simulink model "WorkingModel"  (R2023b)
settings: Solver=FixedStepDiscrete  StartTime=0.0  StopTime=param_sim_time  FixedStep=1/fs  MaxStep=1/fs  RelTol=1e-3
undefined symbols (not defined in the file): analyses, fdesignblkfcn, fs, gcbh, param_tot_samples
libraries: dspstat3 x13, SCGAnalysis_SignalGenerationLib x2
(part 9 of 20)

== system WorkingModel/SCG Analysis/Enabled SCG Analysis Subsystem/All Signals Signal Metric Characterization/SCG Systolic 3DMinS1p2pProjection Signal Metric Characterization/Average Cycle-to-cycle Morphological Variability Calculator ==
  note: This subsystem is only enabled when its signal metric flag is raised.
  in_r_pos : Inport
  in_scg_signal : Inport  Port=2
  Enable : EnablePort
  Average Cycle-to-cycle Morphological Variability Calculator : MATLAB Function  TreatAsAtomicUnit=on
  Constant : Constant  Value=fs
  out_morphological_variability : Outport
  wires:
  Constant/1 -> Average Cycle-to-cycle Morphological Variability Calculator/1(fs)
  Average Cycle-to-cycle Morphological Variability Calculator/1(variability) -> out_morphological_variability/1
  in_scg_signal/1 -> Average Cycle-to-cycle Morphological Variability Calculator/3(scg_signal)
  in_r_pos/1 -> Average Cycle-to-cycle Morphological Variability Calculator/2(r_pos)

== system WorkingModel/SCG Analysis/Enabled SCG Analysis Subsystem/All Signals Signal Metric Characterization/SCG Systolic 3DMinS1p2pProjection Signal Metric Characterization/Average S1 peak-to-peak Amplitude Calculator ==
  note: This subsystem is only enabled when its signal metric flag is raised.
  in_r_pos : Inport
  in_scg_sig : Inport  Port=2
  Enable : EnablePort
  Average S1p2p Amplitude Calculator : MATLAB Function  TreatAsAtomicUnit=on
  Constant : Constant  Value=fs
  out_average_s1p2pamp : Outport
  wires:
  Constant/1 -> Average S1p2p Amplitude Calculator/1(fs)
  in_r_pos/1 -> Average S1p2p Amplitude Calculator/2(r_pos)
  Average S1p2p Amplitude Calculator/1(average_s1p2pamp) -> out_average_s1p2pamp/1
  in_scg_sig/1 -> Average S1p2p Amplitude Calculator/3(scg_signal)

== system WorkingModel/SCG Analysis/Enabled SCG Analysis Subsystem/All Signals Signal Metric Characterization/SCG Systolic 3DMinS1p2pProjection Signal Metric Characterization/Average S2 peak-to-peak Amplitude Calculator ==
  note: This subsystem is only enabled when its signal metric flag is raised.
  in_r_pos : Inport
  in_scg_signal : Inport  Port=2
  Enable : EnablePort
  Average S2p2p Amplitude Calculator : MATLAB Function  TreatAsAtomicUnit=on
  Constant : Constant  Value=fs
  out_scg_signal_average_s2p2pamp : Outport
  wires:
  in_scg_signal/1 -> Average S2p2p Amplitude Calculator/3(scg_signal)
  Average S2p2p Amplitude Calculator/1(average_s2p2pamp) -> out_scg_signal_average_s2p2pamp/1
  in_r_pos/1 -> Average S2p2p Amplitude Calculator/2(r_pos)
  Constant/1 -> Average S2p2p Amplitude Calculator/1(fs)

== system WorkingModel/SCG Analysis/Enabled SCG Analysis Subsystem/All Signals Signal Metric Characterization/SCG Systolic 3DMinS1p2pProjection Signal Metric Characterization/Average Signal-to-Noise Ratio Calculator ==
  note: This subsystem is only enabled when its signal metric flag is raised.
  in_r_pos : Inport
  in_scg_signal : Inport  Port=2
  Enable : EnablePort  PropagateVarSize=During execution
  Average S1 Signal-to-Noise Ratio : Subsystem
  Average S1X Signal-to-Noise Ratio : Subsystem
  Average S2 Signal-to-Noise Ratio : Subsystem
  Average S2X Signal-to-Noise Ratio : Subsystem
  out_scg_signal_average_s1snr : Outport
  out_scg_signal_average_s1Xsnr : Outport  Port=2
  out_scg_signal_average_s2snr : Outport  Port=3
  out_scg_signal_average_s2Xsnr : Outport  Port=4
  wires:
  Average S2X Signal-to-Noise Ratio/1(average_s2Xsnr) -> out_scg_signal_average_s2Xsnr/1
  in_r_pos/1 -> Average S1 Signal-to-Noise Ratio/1(r_pos), Average S2X Signal-to-Noise Ratio/1(r_pos), Average S2 Signal-to-Noise Ratio/1(r_pos), Average S1X Signal-to-Noise Ratio/1(r_pos)
  Average S2 Signal-to-Noise Ratio/1(average_s2snr) -> out_scg_signal_average_s2snr/1
  Average S1X Signal-to-Noise Ratio/1(average_s1Xsnr) -> out_scg_signal_average_s1Xsnr/1
  in_scg_signal/1 -> Average S2X Signal-to-Noise Ratio/2(scg_signal), Average S2 Signal-to-Noise Ratio/2(scg_signal), Average S1X Signal-to-Noise Ratio/2(scg_signal), Average S1 Signal-to-Noise Ratio/2(scg_signal)
  Average S1 Signal-to-Noise Ratio/1(average_s1snr) -> out_scg_signal_average_s1snr/1

== system WorkingModel/SCG Analysis/Enabled SCG Analysis Subsystem/All Signals Signal Metric Characterization/SCG Systolic 3DMinS1p2pProjection Signal Metric Characterization/Spectral Distribution Calculator ==
  note: This subsystem is only enabled when its signal metric flag is raised.
  in_r_pos : Inport
  in_scg_signal : Inport  Port=2
  Enable : EnablePort
  Constant : Constant  Value=fs
  Constant1 : Constant  Value=entire_cycle
  Constant2 : Constant  Value=s1
  Constant3 : Constant  Value=s2
  Constant4 : Constant  Value=f_band_lo
  Constant5 : Constant  Value=f_band_mid
  Constant6 : Constant  Value=f_band_hi
  Spectral Distribution Calculator : MATLAB Function  TreatAsAtomicUnit=on
  out_entire_cycle_spectral_distribution : Outport
  out_s1_spectral_distribution : Outport  Port=2
  out_s2_spectral_distribution : Outport  Port=3
  wires:
  in_r_pos/1 -> Spectral Distribution Calculator/2(r_pos)
  in_scg_signal/1 -> Spectral Distribution Calculator/3(scg_signal)
  Spectral Distribution Calculator/1(entire_cycle_nsd) -> out_entire_cycle_spectral_distribution/1
  Constant/1 -> Spectral Distribution Calculator/1(fs)
  Constant1/1 -> Spectral Distribution Calculator/4(entire_cycle_flag)
  Constant4/1 -> Spectral Distribution Calculator/7(f_band_lo)
  Constant6/1 -> Spectral Distribution Calculator/9(f_band_hi)
  Constant5/1 -> Spectral Distribution Calculator/8(f_band_mid)
  Constant3/1 -> Spectral Distribution Calculator/6(s2_flag)
  Constant2/1 -> Spectral Distribution Calculator/5(s1_flag)
  Spectral Distribution Calculator/3(s2_nsd) -> out_s2_spectral_distribution/1
  Spectral Distribution Calculator/2(s1_nsd) -> out_s1_spectral_distribution/1

== system WorkingModel/SCG Analysis/Enabled SCG Analysis Subsystem/All Signals Signal Metric Characterization/SCG Systolic 3DMinS1p2pProjection Signal Metric Characterization/Variance ==
  note: This subsystem is only enabled when its signal metric flag is raised.
  in_scg_signal : Inport
  Enable : EnablePort
  Variance : dspstat3/Variance  run=off  InputProcessing=Columns as channels (frame based)  reset_popup=None  directionMode=Each column  dimension=1  roiEnable=off  roiType=Rectangles  roiPortion=Entire ROI  roiOutput=Individual statistics for each ROI  roiFlag=off  roundingMode=Floor  overflowMode=off
  out_scg_signal_var : Outport
  wires:
  Variance/1 -> out_scg_signal_var/1
  in_scg_signal/1 -> Variance/1

== system WorkingModel/SCG Analysis/Enabled SCG Analysis Subsystem/All Signals Signal Metric Characterization/SCG X Signal Metric Characterization/Average Cycle-to-cycle Morphological Variability Calculator ==
  note: This subsystem is only enabled when its signal metric flag is raised.
  in_r_pos : Inport
  in_scg_signal : Inport  Port=2
  Enable : EnablePort
  Average Cycle-to-cycle Morphological Variability Calculator : MATLAB Function  TreatAsAtomicUnit=on
  Constant : Constant  Value=fs
  out_morphological_variability : Outport
  wires:
  Constant/1 -> Average Cycle-to-cycle Morphological Variability Calculator/1(fs)
  Average Cycle-to-cycle Morphological Variability Calculator/1(variability) -> out_morphological_variability/1
  in_scg_signal/1 -> Average Cycle-to-cycle Morphological Variability Calculator/3(scg_signal)
  in_r_pos/1 -> Average Cycle-to-cycle Morphological Variability Calculator/2(r_pos)

== system WorkingModel/SCG Analysis/Enabled SCG Analysis Subsystem/All Signals Signal Metric Characterization/SCG X Signal Metric Characterization/Average S1 peak-to-peak Amplitude Calculator ==
  note: This subsystem is only enabled when its signal metric flag is raised.
  in_r_pos : Inport
  in_scg_sig : Inport  Port=2
  Enable : EnablePort
  Average S1p2p Amplitude Calculator : MATLAB Function  TreatAsAtomicUnit=on
  Constant : Constant  Value=fs
  out_average_s1p2pamp : Outport
  wires:
  Constant/1 -> Average S1p2p Amplitude Calculator/1(fs)
  in_r_pos/1 -> Average S1p2p Amplitude Calculator/2(r_pos)
  Average S1p2p Amplitude Calculator/1(average_s1p2pamp) -> out_average_s1p2pamp/1
  in_scg_sig/1 -> Average S1p2p Amplitude Calculator/3(scg_signal)

== system WorkingModel/SCG Analysis/Enabled SCG Analysis Subsystem/All Signals Signal Metric Characterization/SCG X Signal Metric Characterization/Average S2 peak-to-peak Amplitude Calculator ==
  note: This subsystem is only enabled when its signal metric flag is raised.
  in_r_pos : Inport
  in_scg_signal : Inport  Port=2
  Enable : EnablePort
  Average S2p2p Amplitude Calculator : MATLAB Function  TreatAsAtomicUnit=on
  Constant : Constant  Value=fs
  out_scg_signal_average_s2p2pamp : Outport
  wires:
  in_scg_signal/1 -> Average S2p2p Amplitude Calculator/3(scg_signal)
  Average S2p2p Amplitude Calculator/1(average_s2p2pamp) -> out_scg_signal_average_s2p2pamp/1
  in_r_pos/1 -> Average S2p2p Amplitude Calculator/2(r_pos)
  Constant/1 -> Average S2p2p Amplitude Calculator/1(fs)

== system WorkingModel/SCG Analysis/Enabled SCG Analysis Subsystem/All Signals Signal Metric Characterization/SCG X Signal Metric Characterization/Average Signal-to-Noise Ratio Calculator ==
  note: This subsystem is only enabled when its signal metric flag is raised.
  in_r_pos : Inport
  in_scg_signal : Inport  Port=2
  Enable : EnablePort  PropagateVarSize=During execution
  Average S1 Signal-to-Noise Ratio : Subsystem
  Average S1X Signal-to-Noise Ratio : Subsystem
  Average S2 Signal-to-Noise Ratio : Subsystem
  Average S2X Signal-to-Noise Ratio : Subsystem
  out_scg_signal_average_s1snr : Outport
  out_scg_signal_average_s1Xsnr : Outport  Port=2
  out_scg_signal_average_s2snr : Outport  Port=3
  out_scg_signal_average_s2Xsnr : Outport  Port=4
  wires:
  Average S2X Signal-to-Noise Ratio/1(average_s2Xsnr) -> out_scg_signal_average_s2Xsnr/1
  in_r_pos/1 -> Average S1 Signal-to-Noise Ratio/1(r_pos), Average S2X Signal-to-Noise Ratio/1(r_pos), Average S2 Signal-to-Noise Ratio/1(r_pos), Average S1X Signal-to-Noise Ratio/1(r_pos)
  Average S2 Signal-to-Noise Ratio/1(average_s2snr) -> out_scg_signal_average_s2snr/1
  Average S1X Signal-to-Noise Ratio/1(average_s1Xsnr) -> out_scg_signal_average_s1Xsnr/1
  in_scg_signal/1 -> Average S2X Signal-to-Noise Ratio/2(scg_signal), Average S2 Signal-to-Noise Ratio/2(scg_signal), Average S1X Signal-to-Noise Ratio/2(scg_signal), Average S1 Signal-to-Noise Ratio/2(scg_signal)
  Average S1 Signal-to-Noise Ratio/1(average_s1snr) -> out_scg_signal_average_s1snr/1

== system WorkingModel/SCG Analysis/Enabled SCG Analysis Subsystem/All Signals Signal Metric Characterization/SCG X Signal Metric Characterization/Spectral Distribution Calculator ==
  note: This subsystem is only enabled when its signal metric flag is raised.
  in_r_pos : Inport
  in_scg_signal : Inport  Port=2
  Enable : EnablePort
  Constant : Constant  Value=fs
  Constant1 : Constant  Value=entire_cycle
  Constant2 : Constant  Value=s1
  Constant3 : Constant  Value=s2
  Constant4 : Constant  Value=f_band_lo
  Constant5 : Constant  Value=f_band_mid
  Constant6 : Constant  Value=f_band_hi
  Spectral Distribution Calculator : MATLAB Function  TreatAsAtomicUnit=on
  out_entire_cycle_spectral_distribution : Outport
  out_s1_spectral_distribution : Outport  Port=2
  out_s2_spectral_distribution : Outport  Port=3
  wires:
  in_r_pos/1 -> Spectral Distribution Calculator/2(r_pos)
  in_scg_signal/1 -> Spectral Distribution Calculator/3(scg_signal)
  Spectral Distribution Calculator/1(entire_cycle_nsd) -> out_entire_cycle_spectral_distribution/1
  Constant/1 -> Spectral Distribution Calculator/1(fs)
  Constant1/1 -> Spectral Distribution Calculator/4(entire_cycle_flag)
  Constant4/1 -> Spectral Distribution Calculator/7(f_band_lo)
  Constant6/1 -> Spectral Distribution Calculator/9(f_band_hi)
  Constant5/1 -> Spectral Distribution Calculator/8(f_band_mid)
  Constant3/1 -> Spectral Distribution Calculator/6(s2_flag)
  Constant2/1 -> Spectral Distribution Calculator/5(s1_flag)
  Spectral Distribution Calculator/3(s2_nsd) -> out_s2_spectral_distribution/1
  Spectral Distribution Calculator/2(s1_nsd) -> out_s1_spectral_distribution/1

== system WorkingModel/SCG Analysis/Enabled SCG Analysis Subsystem/All Signals Signal Metric Characterization/SCG X Signal Metric Characterization/Variance ==
  note: This subsystem is only enabled when its signal metric flag is raised.
  in_scg_signal : Inport
  Enable : EnablePort
  Variance : dspstat3/Variance  run=off  InputProcessing=Columns as channels (frame based)  reset_popup=None  directionMode=Each column  dimension=1  roiEnable=off  roiType=Rectangles  roiPortion=Entire ROI  roiOutput=Individual statistics for each ROI  roiFlag=off  roundingMode=Floor  overflowMode=off
  out_scg_signal_var : Outport
  wires:
  Variance/1 -> out_scg_signal_var/1
  in_scg_signal/1 -> Variance/1

== system WorkingModel/SCG Analysis/Enabled SCG Analysis Subsystem/All Signals Signal Metric Characterization/SCG Y Signal Metric Characterization/Average Cycle-to-cycle Morphological Variability Calculator ==
  note: This subsystem is only enabled when its signal metric flag is raised.
  in_r_pos : Inport
  in_scg_signal : Inport  Port=2
  Enable : EnablePort
  Average Cycle-to-cycle Morphological Variability Calculator : MATLAB Function  TreatAsAtomicUnit=on
  Constant : Constant  Value=fs
  out_morphological_variability : Outport
  wires:
  in_r_pos/1 -> Average Cycle-to-cycle Morphological Variability Calculator/2(r_pos)
  in_scg_signal/1 -> Average Cycle-to-cycle Morphological Variability Calculator/3(scg_signal)
  Average Cycle-to-cycle Morphological Variability Calculator/1(variability) -> out_morphological_variability/1
  Constant/1 -> Average Cycle-to-cycle Morphological Variability Calculator/1(fs)

== system WorkingModel/SCG Analysis/Enabled SCG Analysis Subsystem/All Signals Signal Metric Characterization/SCG Y Signal Metric Characterization/Average S1 peak-to-peak Amplitude Calculator ==
  note: This subsystem is only enabled when its signal metric flag is raised.
  in_r_pos : Inport
  in_scg_sig : Inport  Port=2
  Enable : EnablePort
  Average S1p2p Amplitude Calculator : MATLAB Function  TreatAsAtomicUnit=on
  Constant : Constant  Value=fs
  out_average_s1p2pamp : Outport
  wires:
  in_scg_sig/1 -> Average S1p2p Amplitude Calculator/3(scg_signal)
  Average S1p2p Amplitude Calculator/1(average_s1p2pamp) -> out_average_s1p2pamp/1
  in_r_pos/1 -> Average S1p2p Amplitude Calculator/2(r_pos)
  Constant/1 -> Average S1p2p Amplitude Calculator/1(fs)

== system WorkingModel/SCG Analysis/Enabled SCG Analysis Subsystem/All Signals Signal Metric Characterization/SCG Y Signal Metric Characterization/Average S2 peak-to-peak Amplitude Calculator ==
  note: This subsystem is only enabled when its signal metric flag is raised.
  in_r_pos : Inport
  in_scg_signal : Inport  Port=2
  Enable : EnablePort
  Average S2p2p Amplitude Calculator : MATLAB Function  TreatAsAtomicUnit=on
  Constant : Constant  Value=fs
  out_scg_signal_average_s2p2pamp : Outport
  wires:
  Constant/1 -> Average S2p2p Amplitude Calculator/1(fs)
  in_r_pos/1 -> Average S2p2p Amplitude Calculator/2(r_pos)
  Average S2p2p Amplitude Calculator/1(average_s2p2pamp) -> out_scg_signal_average_s2p2pamp/1
  in_scg_signal/1 -> Average S2p2p Amplitude Calculator/3(scg_signal)

== system WorkingModel/SCG Analysis/Enabled SCG Analysis Subsystem/All Signals Signal Metric Characterization/SCG Y Signal Metric Characterization/Average Signal-to-Noise Ratio Calculator ==
  note: This subsystem is only enabled when its signal metric flag is raised.
  in_r_pos : Inport
  in_scg_signal : Inport  Port=2
  Enable : EnablePort  PropagateVarSize=During execution
  Average S1 Signal-to-Noise Ratio : Subsystem
  Average S1X Signal-to-Noise Ratio : Subsystem
  Average S2 Signal-to-Noise Ratio : Subsystem
  Average S2X Signal-to-Noise Ratio : Subsystem
  out_scg_signal_average_s1snr : Outport
  out_scg_signal_average_s1Xsnr : Outport  Port=2
  out_scg_signal_average_s2snr : Outport  Port=3
  out_scg_signal_average_s2Xsnr : Outport  Port=4
  wires:
  Average S1 Signal-to-Noise Ratio/1(average_s1snr) -> out_scg_signal_average_s1snr/1
  in_scg_signal/1 -> Average S1 Signal-to-Noise Ratio/2(scg_signal), Average S1X Signal-to-Noise Ratio/2(scg_signal), Average S2 Signal-to-Noise Ratio/2(scg_signal), Average S2X Signal-to-Noise Ratio/2(scg_signal)
  Average S1X Signal-to-Noise Ratio/1(average_s1Xsnr) -> out_scg_signal_average_s1Xsnr/1
  Average S2 Signal-to-Noise Ratio/1(average_s2snr) -> out_scg_signal_average_s2snr/1
  in_r_pos/1 -> Average S1X Signal-to-Noise Ratio/1(r_pos), Average S2 Signal-to-Noise Ratio/1(r_pos), Average S2X Signal-to-Noise Ratio/1(r_pos), Average S1 Signal-to-Noise Ratio/1(r_pos)
  Average S2X Signal-to-Noise Ratio/1(average_s2Xsnr) -> out_scg_signal_average_s2Xsnr/1

== system WorkingModel/SCG Analysis/Enabled SCG Analysis Subsystem/All Signals Signal Metric Characterization/SCG Y Signal Metric Characterization/Spectral Distribution Calculator ==
  note: This subsystem is only enabled when its signal metric flag is raised.
  in_r_pos : Inport
  in_scg_signal : Inport  Port=2
  Enable : EnablePort
  Constant : Constant  Value=fs
  Constant1 : Constant  Value=entire_cycle
  Constant2 : Constant  Value=s1
  Constant3 : Constant  Value=s2
  Constant4 : Constant  Value=f_band_lo
  Constant5 : Constant  Value=f_band_mid
  Constant6 : Constant  Value=f_band_hi
  Spectral Distribution Calculator : MATLAB Function  TreatAsAtomicUnit=on
  out_entire_cycle_spectral_distribution : Outport
  out_s1_spectral_distribution : Outport  Port=2
  out_s2_spectral_distribution : Outport  Port=3
  wires:
  Spectral Distribution Calculator/2(s1_nsd) -> out_s1_spectral_distribution/1
  Spectral Distribution Calculator/3(s2_nsd) -> out_s2_spectral_distribution/1
  Constant2/1 -> Spectral Distribution Calculator/5(s1_flag)
  Constant3/1 -> Spectral Distribution Calculator/6(s2_flag)
  Constant5/1 -> Spectral Distribution Calculator/8(f_band_mid)
  Constant6/1 -> Spectral Distribution Calculator/9(f_band_hi)
  Constant4/1 -> Spectral Distribution Calculator/7(f_band_lo)
  Constant1/1 -> Spectral Distribution Calculator/4(entire_cycle_flag)
  Constant/1 -> Spectral Distribution Calculator/1(fs)
  Spectral Distribution Calculator/1(entire_cycle_nsd) -> out_entire_cycle_spectral_distribution/1
  in_scg_signal/1 -> Spectral Distribution Calculator/3(scg_signal)
  in_r_pos/1 -> Spectral Distribution Calculator/2(r_pos)

== system WorkingModel/SCG Analysis/Enabled SCG Analysis Subsystem/All Signals Signal Metric Characterization/SCG Y Signal Metric Characterization/Variance ==
  note: This subsystem is only enabled when its signal metric flag is raised.
  in_scg_signal : Inport
  Enable : EnablePort
  Variance : dspstat3/Variance  run=off  InputProcessing=Columns as channels (frame based)  reset_popup=None  directionMode=Each column  dimension=1  roiEnable=off  roiType=Rectangles  roiPortion=Entire ROI  roiOutput=Individual statistics for each ROI  roiFlag=off  roundingMode=Floor  overflowMode=off
  out_scg_signal_var : Outport
  wires:
  in_scg_signal/1 -> Variance/1
  Variance/1 -> out_scg_signal_var/1

== system WorkingModel/SCG Analysis/Enabled SCG Analysis Subsystem/All Signals Signal Metric Characterization/SCG Z Signal Metric Characterization/Average Cycle-to-cycle Morphological Variability Calculator ==
  note: This subsystem is only enabled when its signal metric flag is raised.
  in_r_pos : Inport
  in_scg_signal : Inport  Port=2
  Enable : EnablePort
  Average Cycle-to-cycle Morphological Variability Calculator : MATLAB Function  TreatAsAtomicUnit=on
  Constant : Constant  Value=fs
  out_morphological_variability : Outport
  wires:
  Constant/1 -> Average Cycle-to-cycle Morphological Variability Calculator/1(fs)
  Average Cycle-to-cycle Morphological Variability Calculator/1(variability) -> out_morphological_variability/1
  in_scg_signal/1 -> Average Cycle-to-cycle Morphological Variability Calculator/3(scg_signal)
  in_r_pos/1 -> Average Cycle-to-cycle Morphological Variability Calculator/2(r_pos)

== system WorkingModel/SCG Analysis/Enabled SCG Analysis Subsystem/All Signals Signal Metric Characterization/SCG Z Signal Metric Characterization/Average S1 peak-to-peak Amplitude Calculator ==
  note: This subsystem is only enabled when its signal metric flag is raised.
  in_r_pos : Inport
  in_scg_sig : Inport  Port=2
  Enable : EnablePort
  Average S1p2p Amplitude Calculator : MATLAB Function  TreatAsAtomicUnit=on
  Constant : Constant  Value=fs
  out_average_s1p2pamp : Outport
  wires:
  Constant/1 -> Average S1p2p Amplitude Calculator/1(fs)
  in_r_pos/1 -> Average S1p2p Amplitude Calculator/2(r_pos)
  Average S1p2p Amplitude Calculator/1(average_s1p2pamp) -> out_average_s1p2pamp/1
  in_scg_sig/1 -> Average S1p2p Amplitude Calculator/3(scg_signal)

== system WorkingModel/SCG Analysis/Enabled SCG Analysis Subsystem/All Signals Signal Metric Characterization/SCG Z Signal Metric Characterization/Average S2 peak-to-peak Amplitude Calculator ==
  note: This subsystem is only enabled when its signal metric flag is raised.
  in_r_pos : Inport
  in_scg_signal : Inport  Port=2
  Enable : EnablePort
  Average S2p2p Amplitude Calculator : MATLAB Function  TreatAsAtomicUnit=on
  Constant : Constant  Value=fs
  out_scg_signal_average_s2p2pamp : Outport
  wires:
  in_scg_signal/1 -> Average S2p2p Amplitude Calculator/3(scg_signal)
  Average S2p2p Amplitude Calculator/1(average_s2p2pamp) -> out_scg_signal_average_s2p2pamp/1
  in_r_pos/1 -> Average S2p2p Amplitude Calculator/2(r_pos)
  Constant/1 -> Average S2p2p Amplitude Calculator/1(fs)

== system WorkingModel/SCG Analysis/Enabled SCG Analysis Subsystem/All Signals Signal Metric Characterization/SCG Z Signal Metric Characterization/Average Signal-to-Noise Ratio Calculator ==
  note: This subsystem is only enabled when its signal metric flag is raised.
  in_r_pos : Inport
  in_scg_signal : Inport  Port=2
  Enable : EnablePort  PropagateVarSize=During execution
  Average S1 Signal-to-Noise Ratio : Subsystem
  Average S1X Signal-to-Noise Ratio : Subsystem
  Average S2 Signal-to-Noise Ratio : Subsystem
  Average S2X Signal-to-Noise Ratio : Subsystem
  out_scg_signal_average_s1snr : Outport
  out_scg_signal_average_s1Xsnr : Outport  Port=2
  out_scg_signal_average_s2snr : Outport  Port=3
  out_scg_signal_average_s2Xsnr : Outport  Port=4
  wires:
  Average S2X Signal-to-Noise Ratio/1(average_s2Xsnr) -> out_scg_signal_average_s2Xsnr/1
  in_r_pos/1 -> Average S1 Signal-to-Noise Ratio/1(r_pos), Average S2X Signal-to-Noise Ratio/1(r_pos), Average S2 Signal-to-Noise Ratio/1(r_pos), Average S1X Signal-to-Noise Ratio/1(r_pos)
  Average S2 Signal-to-Noise Ratio/1(average_s2snr) -> out_scg_signal_average_s2snr/1
  Average S1X Signal-to-Noise Ratio/1(average_s1Xsnr) -> out_scg_signal_average_s1Xsnr/1
  in_scg_signal/1 -> Average S2X Signal-to-Noise Ratio/2(scg_signal), Average S2 Signal-to-Noise Ratio/2(scg_signal), Average S1X Signal-to-Noise Ratio/2(scg_signal), Average S1 Signal-to-Noise Ratio/2(scg_signal)
  Average S1 Signal-to-Noise Ratio/1(average_s1snr) -> out_scg_signal_average_s1snr/1

== system WorkingModel/SCG Analysis/Enabled SCG Analysis Subsystem/All Signals Signal Metric Characterization/SCG Z Signal Metric Characterization/Spectral Distribution Calculator ==
  note: This subsystem is only enabled when its signal metric flag is raised.
  in_r_pos : Inport
  in_scg_signal : Inport  Port=2
  Enable : EnablePort
  Constant : Constant  Value=fs
  Constant1 : Constant  Value=entire_cycle
  Constant2 : Constant  Value=s1
  Constant3 : Constant  Value=s2
  Constant4 : Constant  Value=f_band_lo
  Constant5 : Constant  Value=f_band_mid
  Constant6 : Constant  Value=f_band_hi
  Spectral Distribution Calculator : MATLAB Function  TreatAsAtomicUnit=on
  out_entire_cycle_spectral_distribution : Outport
  out_s1_spectral_distribution : Outport  Port=2
  out_s2_spectral_distribution : Outport  Port=3
  wires:
  in_r_pos/1 -> Spectral Distribution Calculator/2(r_pos)
  in_scg_signal/1 -> Spectral Distribution Calculator/3(scg_signal)
  Spectral Distribution Calculator/1(entire_cycle_nsd) -> out_entire_cycle_spectral_distribution/1
  Constant/1 -> Spectral Distribution Calculator/1(fs)
  Constant1/1 -> Spectral Distribution Calculator/4(entire_cycle_flag)
  Constant4/1 -> Spectral Distribution Calculator/7(f_band_lo)
  Constant6/1 -> Spectral Distribution Calculator/9(f_band_hi)
  Constant5/1 -> Spectral Distribution Calculator/8(f_band_mid)
  Constant3/1 -> Spectral Distribution Calculator/6(s2_flag)
  Constant2/1 -> Spectral Distribution Calculator/5(s1_flag)
  Spectral Distribution Calculator/3(s2_nsd) -> out_s2_spectral_distribution/1
  Spectral Distribution Calculator/2(s1_nsd) -> out_s1_spectral_distribution/1

== system WorkingModel/SCG Analysis/Enabled SCG Analysis Subsystem/All Signals Signal Metric Characterization/SCG Z Signal Metric Characterization/Variance ==
  note: This subsystem is only enabled when its signal metric flag is raised.
  in_scg_signal : Inport
  Enable : EnablePort
  Variance : dspstat3/Variance  run=off  InputProcessing=Columns as channels (frame based)  reset_popup=None  directionMode=Each column  dimension=1  roiEnable=off  roiType=Rectangles  roiPortion=Entire ROI  roiOutput=Individual statistics for each ROI  roiFlag=off  roundingMode=Floor  overflowMode=off
  out_scg_signal_var : Outport
  wires:
  Variance/1 -> out_scg_signal_var/1
  in_scg_signal/1 -> Variance/1

== system WorkingModel/SCG Analysis/Enabled SCG Analysis Subsystem/Signal Generation/2DMod Calculator/2DMod Calculator ==
  2D Components : Inport
  Square Root1 : Sqrt
  Square1 : Math  Operator=square  SignedPower=on
  Sum1 : Sum  Inputs=+  CollapseMode=Specified dimension  CollapseDim=2
  2D Modulus : Outport  VectorParamsAs1DForOutWhenUnconnected=off
  wires:
  Square1/1 -> Sum1/1
  Sum1/1 -> Square Root1/1
  2D Components/1 -> Square1/1
  Square Root1/1 -> 2D Modulus/1

== system WorkingModel/SCG Analysis/Enabled SCG Analysis Subsystem/Signal Generation/3D Projections/3D Max S2 p2p Axis Calculator ==
  avg_scg_xyz_s2 : Inport
  Max S2 P2P  Axis Finder 3D : MATLABFcn  MATLABFcn=cardiac_max_s2p2p_axis_finder_3D  OutputDimensions=4  Output1D=off
  Selector2 : Selector  InputPortWidth=4  IndexOptions=Index vector (dialog)  Indices=[1]  OutputSizes=1
  Selector3 : Selector  InputPortWidth=4  IndexOptions=Index vector (dialog)  Indices=[2]  OutputSizes=1
  Selector6 : Selector  InputPortWidth=4  IndexOptions=Index vector (dialog)  Indices=[3]  OutputSizes=1
  Selector7 : Selector  InputPortWidth=4  IndexOptions=Index vector (dialog)  Indices=[4]  OutputSizes=1
  out_max_s2_axis_elevation : Outport
  out_max_s2_axis_azimuth : Outport  Port=2
  out_min_s2_axis_elevation : Outport  Port=3
  out_min_s2_axis_azimuth : Outport  Port=4
  wires:
  avg_scg_xyz_s2/1 -> Max S2 P2P  Axis Finder 3D/1
  Max S2 P2P  Axis Finder 3D/1 -> Selector7/1, Selector6/1, Selector2/1, Selector3/1
  Selector2/1 -> out_max_s2_axis_elevation/1
  Selector3/1 -> out_max_s2_axis_azimuth/1
  Selector7/1 -> out_min_s2_axis_azimuth/1
  Selector6/1 -> out_min_s2_axis_elevation/1

== system WorkingModel/SCG Analysis/Enabled SCG Analysis Subsystem/Signal Generation/3D Projections/3D S2 Mechanical Axis Calculator ==
  in_avg_scg_xyz_s2 : Inport
  Cardiac Mechanical Diastolic Axis Finder 3D : MATLABFcn  MATLABFcn=cardiac_mech_diastolic_axis_finder_3D  OutputDimensions=4  Output1D=off
  Selector : Selector  InputPortWidth=4  IndexOptions=Index vector (dialog)  Indices=[1]  OutputSizes=1
  Selector1 : Selector  InputPortWidth=4  IndexOptions=Index vector (dialog)  Indices=[2]  OutputSizes=1
  Selector4 : Selector  InputPortWidth=4  IndexOptions=Index vector (dialog)  Indices=[3]  OutputSizes=1
  Selector5 : Selector  InputPortWidth=4  IndexOptions=Index vector (dialog)  Indices=[4]  OutputSizes=1
  out_s2_mech_axis_elevation : Outport
  out_s2_mech_axis_azimuth : Outport  Port=2
  out_s2_antimech_axis_elevation : Outport  Port=3
  out_s2_antimech_axis_azimuth : Outport  Port=4
  wires:
  in_avg_scg_xyz_s2/1 -> Cardiac Mechanical Diastolic Axis Finder 3D/1
  Selector1/1 -> out_s2_mech_axis_azimuth/1
  Selector4/1 -> out_s2_antimech_axis_elevation/1
  Selector/1 -> out_s2_mech_axis_elevation/1
  Selector5/1 -> out_s2_antimech_axis_azimuth/1
  Cardiac Mechanical Diastolic Axis Finder 3D/1 -> Selector1/1, Selector/1, Selector4/1, Selector5/1

== system WorkingModel/SCG Analysis/Enabled SCG Analysis Subsystem/Signal Generation/3D Projections/SCG xyz Average Cycle ==
  in_ecg_r : Inport
  in_scg_xyz : Inport  Port=2
  Average SCGxyz Cycle Calculator : MATLAB Function  TreatAsAtomicUnit=on
  Constant : Constant
  Fixed-Size Converter 2 : Selector  NumberOfDimensions=2  IndexOptions=Starting and ending indices (port),Index vector (dialog)  Indices=[1:min(analyses.ecg.RR)],[1 2 3]  OutputSizes=1,1
  Min RR Calculator : MATLAB Function  TreatAsAtomicUnit=on
  Mux : Mux  Inputs=2
  out_scg_xyz_avgcycle : Outport  VectorParamsAs1DForOutWhenUnconnected=off
  wires:
  in_scg_xyz/1 -> Average SCGxyz Cycle Calculator/2(scgxyz)
  in_ecg_r/1 -> Min RR Calculator/1(r_pos), Average SCGxyz Cycle Calculator/1(r_pos)
  Average SCGxyz Cycle Calculator/1(scgxyz_avgcycle) -> Fixed-Size Converter 2/1
  Fixed-Size Converter 2/1 -> out_scg_xyz_avgcycle/1
  Constant/1 -> Mux/1
  Min RR Calculator/1(min_rr) -> Mux/2
  Mux/1 -> Fixed-Size Converter 2/2

== system WorkingModel/SCG Analysis/Enabled SCG Analysis Subsystem/All Signals Signal Metric Characterization/SCG 2D Mod Signal Metric Characterization/Average Signal-to-Noise Ratio Calculator/Average S1 Signal-to-Noise Ratio ==
  r_pos : Inport
  scg_signal : Inport  Port=2
  " " : Constant  Value=s1snr_flag
  Average S1 SNR Calculator : MATLAB Function  TreatAsAtomicUnit=on
  Constant : Constant  Value=fs
  Constant1 : Constant  Value=0
  Switch : Switch  Criteria=u2 > Threshold  AllowDiffInputSizes=on  SaturateOnIntegerOverflow=off  InputSameDT=off
  average_s1snr : Outport
  wires:
  scg_signal/1 -> Average S1 SNR Calculator/3(scg_signal)
  Average S1 SNR Calculator/1(average_s1_snr) -> average_s1snr/1
  Constant/1 -> Average S1 SNR Calculator/1(fs)
  " "/1 -> Switch/2
  Switch/1 -> Average S1 SNR Calculator/2(r_pos)
  r_pos/1 -> Switch/1
  Constant1/1 -> Switch/3

== system WorkingModel/SCG Analysis/Enabled SCG Analysis Subsystem/All Signals Signal Metric Characterization/SCG 2D Mod Signal Metric Characterization/Average Signal-to-Noise Ratio Calculator/Average S1X Signal-to-Noise Ratio ==
  r_pos : Inport
  scg_signal : Inport  Port=2
  " " : Constant  Value=s1xsnr_flag
  Average S1 SNR Amplitude Calculator : MATLAB Function  TreatAsAtomicUnit=on
  Constant : Constant  Value=fs
  Constant1 : Constant  Value=0
  Switch : Switch  Criteria=u2 > Threshold  AllowDiffInputSizes=on  SaturateOnIntegerOverflow=off  InputSameDT=off
  average_s1Xsnr : Outport
  wires:
  Average S1 SNR Amplitude Calculator/1(average_s1x_snr) -> average_s1Xsnr/1
  Switch/1 -> Average S1 SNR Amplitude Calculator/2(r_pos)
  scg_signal/1 -> Average S1 SNR Amplitude Calculator/3(scg_signal)
  Constant/1 -> Average S1 SNR Amplitude Calculator/1(fs)
  " "/1 -> Switch/2
  Constant1/1 -> Switch/3
  r_pos/1 -> Switch/1

== system WorkingModel/SCG Analysis/Enabled SCG Analysis Subsystem/All Signals Signal Metric Characterization/SCG 2D Mod Signal Metric Characterization/Average Signal-to-Noise Ratio Calculator/Average S2 Signal-to-Noise Ratio ==
  r_pos : Inport
  scg_signal : Inport  Port=2
  " " : Constant  Value=s2snr_flag
  Average S2 SNR Calculator : MATLAB Function  TreatAsAtomicUnit=on
  Constant : Constant  Value=fs
  Constant1 : Constant  Value=0
  Switch : Switch  Criteria=u2 > Threshold  AllowDiffInputSizes=on  SaturateOnIntegerOverflow=off  InputSameDT=off
  average_s2snr : Outport
  wires:
  Average S2 SNR Calculator/1(average_s2_snr) -> average_s2snr/1
  Switch/1 -> Average S2 SNR Calculator/2(r_pos)
  scg_signal/1 -> Average S2 SNR Calculator/3(scg_signal)
  Constant/1 -> Average S2 SNR Calculator/1(fs)
  " "/1 -> Switch/2
  Constant1/1 -> Switch/3
  r_pos/1 -> Switch/1

== system WorkingModel/SCG Analysis/Enabled SCG Analysis Subsystem/All Signals Signal Metric Characterization/SCG 2D Mod Signal Metric Characterization/Average Signal-to-Noise Ratio Calculator/Average S2X Signal-to-Noise Ratio ==
  r_pos : Inport
  scg_signal : Inport  Port=2
  " " : Constant  Value=s2xsnr_flag
  Average S2X SNR Calculator : MATLAB Function  TreatAsAtomicUnit=on
  Constant : Constant  Value=fs
  Constant1 : Constant  Value=0
  Switch : Switch  Criteria=u2 > Threshold  AllowDiffInputSizes=on  SaturateOnIntegerOverflow=off  InputSameDT=off
  average_s2Xsnr : Outport
  wires:
  Average S2X SNR Calculator/1(average_s2x_snr) -> average_s2Xsnr/1
  Switch/1 -> Average S2X SNR Calculator/2(r_pos)
  scg_signal/1 -> Average S2X SNR Calculator/3(scg_signal)
  Constant/1 -> Average S2X SNR Calculator/1(fs)
  " "/1 -> Switch/2
  Constant1/1 -> Switch/3
  r_pos/1 -> Switch/1

== system WorkingModel/SCG Analysis/Enabled SCG Analysis Subsystem/All Signals Signal Metric Characterization/SCG 3D Mod Signal Metric Characterization/Average Signal-to-Noise Ratio Calculator/Average S1 Signal-to-Noise Ratio ==
  r_pos : Inport
  scg_signal : Inport  Port=2
  " " : Constant  Value=s1snr_flag
  Average S1 SNR Calculator : MATLAB Function  TreatAsAtomicUnit=on
  Constant : Constant  Value=fs
  Constant1 : Constant  Value=0
  Switch : Switch  Criteria=u2 > Threshold  AllowDiffInputSizes=on  SaturateOnIntegerOverflow=off  InputSameDT=off
  average_s1snr : Outport
  wires:
  Constant1/1 -> Switch/3
  r_pos/1 -> Switch/1
  Switch/1 -> Average S1 SNR Calculator/2(r_pos)
  " "/1 -> Switch/2
  Constant/1 -> Average S1 SNR Calculator/1(fs)
  Average S1 SNR Calculator/1(average_s1_snr) -> average_s1snr/1
  scg_signal/1 -> Average S1 SNR Calculator/3(scg_signal)

== system WorkingModel/SCG Analysis/Enabled SCG Analysis Subsystem/All Signals Signal Metric Characterization/SCG 3D Mod Signal Metric Characterization/Average Signal-to-Noise Ratio Calculator/Average S1X Signal-to-Noise Ratio ==
  r_pos : Inport
  scg_signal : Inport  Port=2
  " " : Constant  Value=s1xsnr_flag
  Average S1 SNR Amplitude Calculator : MATLAB Function  TreatAsAtomicUnit=on
  Constant : Constant  Value=fs
  Constant1 : Constant  Value=0
  Switch : Switch  Criteria=u2 > Threshold  AllowDiffInputSizes=on  SaturateOnIntegerOverflow=off  InputSameDT=off
  average_s1Xsnr : Outport
  wires:
  r_pos/1 -> Switch/1
  Constant1/1 -> Switch/3
  " "/1 -> Switch/2
  Constant/1 -> Average S1 SNR Amplitude Calculator/1(fs)
  scg_signal/1 -> Average S1 SNR Amplitude Calculator/3(scg_signal)
  Switch/1 -> Average S1 SNR Amplitude Calculator/2(r_pos)
  Average S1 SNR Amplitude Calculator/1(average_s1x_snr) -> average_s1Xsnr/1

== system WorkingModel/SCG Analysis/Enabled SCG Analysis Subsystem/All Signals Signal Metric Characterization/SCG 3D Mod Signal Metric Characterization/Average Signal-to-Noise Ratio Calculator/Average S2 Signal-to-Noise Ratio ==
  r_pos : Inport
  scg_signal : Inport  Port=2
  " " : Constant  Value=s2snr_flag
  Average S2 SNR Calculator : MATLAB Function  TreatAsAtomicUnit=on
  Constant : Constant  Value=fs
  Constant1 : Constant  Value=0
  Switch : Switch  Criteria=u2 > Threshold  AllowDiffInputSizes=on  SaturateOnIntegerOverflow=off  InputSameDT=off
  average_s2snr : Outport
  wires:
  r_pos/1 -> Switch/1
  Constant1/1 -> Switch/3
  " "/1 -> Switch/2
  Constant/1 -> Average S2 SNR Calculator/1(fs)
  scg_signal/1 -> Average S2 SNR Calculator/3(scg_signal)
  Switch/1 -> Average S2 SNR Calculator/2(r_pos)
  Average S2 SNR Calculator/1(average_s2_snr) -> average_s2snr/1

== system WorkingModel/SCG Analysis/Enabled SCG Analysis Subsystem/All Signals Signal Metric Characterization/SCG 3D Mod Signal Metric Characterization/Average Signal-to-Noise Ratio Calculator/Average S2X Signal-to-Noise Ratio ==
  r_pos : Inport
  scg_signal : Inport  Port=2
  " " : Constant  Value=s2xsnr_flag
  Average S2X SNR Calculator : MATLAB Function  TreatAsAtomicUnit=on
  Constant : Constant  Value=fs
  Constant1 : Constant  Value=0
  Switch : Switch  Criteria=u2 > Threshold  AllowDiffInputSizes=on  SaturateOnIntegerOverflow=off  InputSameDT=off
  average_s2Xsnr : Outport
  wires:
  r_pos/1 -> Switch/1
  Constant1/1 -> Switch/3
  " "/1 -> Switch/2
  Constant/1 -> Average S2X SNR Calculator/1(fs)
  scg_signal/1 -> Average S2X SNR Calculator/3(scg_signal)
  Switch/1 -> Average S2X SNR Calculator/2(r_pos)
  Average S2X SNR Calculator/1(average_s2x_snr) -> average_s2Xsnr/1

== system WorkingModel/SCG Analysis/Enabled SCG Analysis Subsystem/All Signals Signal Metric Characterization/SCG 3DMaxS2p2pProjection Signal Metric Characterization/Average Signal-to-Noise Ratio Calculator/Average S1 Signal-to-Noise Ratio ==
  r_pos : Inport
  scg_signal : Inport  Port=2
  " " : Constant  Value=s1snr_flag
  Average S1 SNR Calculator : MATLAB Function  TreatAsAtomicUnit=on
  Constant : Constant  Value=fs
  Constant1 : Constant  Value=0
  Switch : Switch  Criteria=u2 > Threshold  AllowDiffInputSizes=on  SaturateOnIntegerOverflow=off  InputSameDT=off
  average_s1snr : Outport
  wires:
  Constant1/1 -> Switch/3
  r_pos/1 -> Switch/1
  Switch/1 -> Average S1 SNR Calculator/2(r_pos)
  " "/1 -> Switch/2
  Constant/1 -> Average S1 SNR Calculator/1(fs)
  Average S1 SNR Calculator/1(average_s1_snr) -> average_s1snr/1
  scg_signal/1 -> Average S1 SNR Calculator/3(scg_signal)

== system WorkingModel/SCG Analysis/Enabled SCG Analysis Subsystem/All Signals Signal Metric Characterization/SCG 3DMaxS2p2pProjection Signal Metric Characterization/Average Signal-to-Noise Ratio Calculator/Average S1X Signal-to-Noise Ratio ==
  r_pos : Inport
  scg_signal : Inport  Port=2
  " " : Constant  Value=s1xsnr_flag
  Average S1 SNR Amplitude Calculator : MATLAB Function  TreatAsAtomicUnit=on
  Constant : Constant  Value=fs
  Constant1 : Constant  Value=0
  Switch : Switch  Criteria=u2 > Threshold  AllowDiffInputSizes=on  SaturateOnIntegerOverflow=off  InputSameDT=off
  average_s1Xsnr : Outport
  wires:
  r_pos/1 -> Switch/1
  Constant1/1 -> Switch/3
  " "/1 -> Switch/2
  Constant/1 -> Average S1 SNR Amplitude Calculator/1(fs)
  scg_signal/1 -> Average S1 SNR Amplitude Calculator/3(scg_signal)
  Switch/1 -> Average S1 SNR Amplitude Calculator/2(r_pos)
  Average S1 SNR Amplitude Calculator/1(average_s1x_snr) -> average_s1Xsnr/1

== system WorkingModel/SCG Analysis/Enabled SCG Analysis Subsystem/All Signals Signal Metric Characterization/SCG 3DMaxS2p2pProjection Signal Metric Characterization/Average Signal-to-Noise Ratio Calculator/Average S2 Signal-to-Noise Ratio ==
  r_pos : Inport
  scg_signal : Inport  Port=2
  " " : Constant  Value=s2snr_flag
  Average S2 SNR Calculator : MATLAB Function  TreatAsAtomicUnit=on
  Constant : Constant  Value=fs
  Constant1 : Constant  Value=0
  Switch : Switch  Criteria=u2 > Threshold  AllowDiffInputSizes=on  SaturateOnIntegerOverflow=off  InputSameDT=off
  average_s2snr : Outport
  wires:
  r_pos/1 -> Switch/1
  Constant1/1 -> Switch/3
  " "/1 -> Switch/2
  Constant/1 -> Average S2 SNR Calculator/1(fs)
  scg_signal/1 -> Average S2 SNR Calculator/3(scg_signal)
  Switch/1 -> Average S2 SNR Calculator/2(r_pos)
  Average S2 SNR Calculator/1(average_s2_snr) -> average_s2snr/1

== system WorkingModel/SCG Analysis/Enabled SCG Analysis Subsystem/All Signals Signal Metric Characterization/SCG 3DMaxS2p2pProjection Signal Metric Characterization/Average Signal-to-Noise Ratio Calculator/Average S2X Signal-to-Noise Ratio ==
  r_pos : Inport
  scg_signal : Inport  Port=2
  " " : Constant  Value=s2xsnr_flag
  Average S2X SNR Calculator : MATLAB Function  TreatAsAtomicUnit=on
  Constant : Constant  Value=fs
  Constant1 : Constant  Value=0
  Switch : Switch  Criteria=u2 > Threshold  AllowDiffInputSizes=on  SaturateOnIntegerOverflow=off  InputSameDT=off
  average_s2Xsnr : Outport
  wires:
  r_pos/1 -> Switch/1
  Constant1/1 -> Switch/3
  " "/1 -> Switch/2
  Constant/1 -> Average S2X SNR Calculator/1(fs)
  scg_signal/1 -> Average S2X SNR Calculator/3(scg_signal)
  Switch/1 -> Average S2X SNR Calculator/2(r_pos)
  Average S2X SNR Calculator/1(average_s2x_snr) -> average_s2Xsnr/1

== system WorkingModel/SCG Analysis/Enabled SCG Analysis Subsystem/All Signals Signal Metric Characterization/SCG 3DMinS2p2pProjection Signal Metric Characterization/Average Signal-to-Noise Ratio Calculator/Average S1 Signal-to-Noise Ratio ==
  r_pos : Inport
  scg_signal : Inport  Port=2
  " " : Constant  Value=s1snr_flag
  Average S1 SNR Calculator : MATLAB Function  TreatAsAtomicUnit=on
  Constant : Constant  Value=fs
  Constant1 : Constant  Value=0
  Switch : Switch  Criteria=u2 > Threshold  AllowDiffInputSizes=on  SaturateOnIntegerOverflow=off  InputSameDT=off
  average_s1snr : Outport
  wires:
  scg_signal/1 -> Average S1 SNR Calculator/3(scg_signal)
  Average S1 SNR Calculator/1(average_s1_snr) -> average_s1snr/1
  Constant/1 -> Average S1 SNR Calculator/1(fs)
  " "/1 -> Switch/2
  Switch/1 -> Average S1 SNR Calculator/2(r_pos)
  r_pos/1 -> Switch/1
  Constant1/1 -> Switch/3

== system WorkingModel/SCG Analysis/Enabled SCG Analysis Subsystem/All Signals Signal Metric Characterization/SCG 3DMinS2p2pProjection Signal Metric Characterization/Average Signal-to-Noise Ratio Calculator/Average S1X Signal-to-Noise Ratio ==
  r_pos : Inport
  scg_signal : Inport  Port=2
  " " : Constant  Value=s1xsnr_flag
  Average S1 SNR Amplitude Calculator : MATLAB Function  TreatAsAtomicUnit=on
  Constant : Constant  Value=fs
  Constant1 : Constant  Value=0
  Switch : Switch  Criteria=u2 > Threshold  AllowDiffInputSizes=on  SaturateOnIntegerOverflow=off  InputSameDT=off
  average_s1Xsnr : Outport
  wires:
  Average S1 SNR Amplitude Calculator/1(average_s1x_snr) -> average_s1Xsnr/1
  Switch/1 -> Average S1 SNR Amplitude Calculator/2(r_pos)
  scg_signal/1 -> Average S1 SNR Amplitude Calculator/3(scg_signal)
  Constant/1 -> Average S1 SNR Amplitude Calculator/1(fs)
  " "/1 -> Switch/2
  Constant1/1 -> Switch/3
  r_pos/1 -> Switch/1

== system WorkingModel/SCG Analysis/Enabled SCG Analysis Subsystem/All Signals Signal Metric Characterization/SCG 3DMinS2p2pProjection Signal Metric Characterization/Average Signal-to-Noise Ratio Calculator/Average S2 Signal-to-Noise Ratio ==
  r_pos : Inport
  scg_signal : Inport  Port=2
  " " : Constant  Value=s2snr_flag
  Average S2 SNR Calculator : MATLAB Function  TreatAsAtomicUnit=on
  Constant : Constant  Value=fs
  Constant1 : Constant  Value=0
  Switch : Switch  Criteria=u2 > Threshold  AllowDiffInputSizes=on  SaturateOnIntegerOverflow=off  InputSameDT=off
  average_s2snr : Outport
  wires:
  Average S2 SNR Calculator/1(average_s2_snr) -> average_s2snr/1
  Switch/1 -> Average S2 SNR Calculator/2(r_pos)
  scg_signal/1 -> Average S2 SNR Calculator/3(scg_signal)
  Constant/1 -> Average S2 SNR Calculator/1(fs)
  " "/1 -> Switch/2
  Constant1/1 -> Switch/3
  r_pos/1 -> Switch/1

== system WorkingModel/SCG Analysis/Enabled SCG Analysis Subsystem/All Signals Signal Metric Characterization/SCG 3DMinS2p2pProjection Signal Metric Characterization/Average Signal-to-Noise Ratio Calculator/Average S2X Signal-to-Noise Ratio ==
  r_pos : Inport
  scg_signal : Inport  Port=2
  " " : Constant  Value=s2xsnr_flag
  Average S2X SNR Calculator : MATLAB Function  TreatAsAtomicUnit=on
  Constant : Constant  Value=fs
  Constant1 : Constant  Value=0
  Switch : Switch  Criteria=u2 > Threshold  AllowDiffInputSizes=on  SaturateOnIntegerOverflow=off  InputSameDT=off
  average_s2Xsnr : Outport
  wires:
  Average S2X SNR Calculator/1(average_s2x_snr) -> average_s2Xsnr/1
  Switch/1 -> Average S2X SNR Calculator/2(r_pos)
  scg_signal/1 -> Average S2X SNR Calculator/3(scg_signal)
  Constant/1 -> Average S2X SNR Calculator/1(fs)
  " "/1 -> Switch/2
  Constant1/1 -> Switch/3
  r_pos/1 -> Switch/1

== system WorkingModel/SCG Analysis/Enabled SCG Analysis Subsystem/All Signals Signal Metric Characterization/SCG S2 3DAntiMechAxis Signal Metric Characterization/Average Signal-to-Noise Ratio Calculator/Average S1 Signal-to-Noise Ratio ==
  r_pos : Inport
  scg_signal : Inport  Port=2
  " " : Constant  Value=s1snr_flag
  Average S1 SNR Calculator : MATLAB Function  TreatAsAtomicUnit=on
  Constant : Constant  Value=fs
  Constant1 : Constant  Value=0
  Switch : Switch  Criteria=u2 > Threshold  AllowDiffInputSizes=on  SaturateOnIntegerOverflow=off  InputSameDT=off
  average_s1snr : Outport
  wires:
  scg_signal/1 -> Average S1 SNR Calculator/3(scg_signal)
  Average S1 SNR Calculator/1(average_s1_snr) -> average_s1snr/1
  Constant/1 -> Average S1 SNR Calculator/1(fs)
  " "/1 -> Switch/2
  Switch/1 -> Average S1 SNR Calculator/2(r_pos)
  r_pos/1 -> Switch/1
  Constant1/1 -> Switch/3

== system WorkingModel/SCG Analysis/Enabled SCG Analysis Subsystem/All Signals Signal Metric Characterization/SCG S2 3DAntiMechAxis Signal Metric Characterization/Average Signal-to-Noise Ratio Calculator/Average S1X Signal-to-Noise Ratio ==
  r_pos : Inport
  scg_signal : Inport  Port=2
  " " : Constant  Value=s1xsnr_flag
  Average S1 SNR Amplitude Calculator : MATLAB Function  TreatAsAtomicUnit=on
  Constant : Constant  Value=fs
  Constant1 : Constant  Value=0
  Switch : Switch  Criteria=u2 > Threshold  AllowDiffInputSizes=on  SaturateOnIntegerOverflow=off  InputSameDT=off
  average_s1Xsnr : Outport
  wires:
  Average S1 SNR Amplitude Calculator/1(average_s1x_snr) -> average_s1Xsnr/1
  Switch/1 -> Average S1 SNR Amplitude Calculator/2(r_pos)
  scg_signal/1 -> Average S1 SNR Amplitude Calculator/3(scg_signal)
  Constant/1 -> Average S1 SNR Amplitude Calculator/1(fs)
  " "/1 -> Switch/2
  Constant1/1 -> Switch/3
  r_pos/1 -> Switch/1

== system WorkingModel/SCG Analysis/Enabled SCG Analysis Subsystem/All Signals Signal Metric Characterization/SCG S2 3DAntiMechAxis Signal Metric Characterization/Average Signal-to-Noise Ratio Calculator/Average S2 Signal-to-Noise Ratio ==
  r_pos : Inport
  scg_signal : Inport  Port=2
  " " : Constant  Value=s2snr_flag
  Average S2 SNR Calculator : MATLAB Function  TreatAsAtomicUnit=on
  Constant : Constant  Value=fs
  Constant1 : Constant  Value=0
  Switch : Switch  Criteria=u2 > Threshold  AllowDiffInputSizes=on  SaturateOnIntegerOverflow=off  InputSameDT=off
  average_s2snr : Outport
  wires:
  Average S2 SNR Calculator/1(average_s2_snr) -> average_s2snr/1
  Switch/1 -> Average S2 SNR Calculator/2(r_pos)
  scg_signal/1 -> Average S2 SNR Calculator/3(scg_signal)
  Constant/1 -> Average S2 SNR Calculator/1(fs)
  " "/1 -> Switch/2
  Constant1/1 -> Switch/3
  r_pos/1 -> Switch/1

== system WorkingModel/SCG Analysis/Enabled SCG Analysis Subsystem/All Signals Signal Metric Characterization/SCG S2 3DAntiMechAxis Signal Metric Characterization/Average Signal-to-Noise Ratio Calculator/Average S2X Signal-to-Noise Ratio ==
  r_pos : Inport
  scg_signal : Inport  Port=2
  " " : Constant  Value=s2xsnr_flag
  Average S2X SNR Calculator : MATLAB Function  TreatAsAtomicUnit=on
  Constant : Constant  Value=fs
  Constant1 : Constant  Value=0
  Switch : Switch  Criteria=u2 > Threshold  AllowDiffInputSizes=on  SaturateOnIntegerOverflow=off  InputSameDT=off
  average_s2Xsnr : Outport
  wires:
  Average S2X SNR Calculator/1(average_s2x_snr) -> average_s2Xsnr/1
  Switch/1 -> Average S2X SNR Calculator/2(r_pos)
  scg_signal/1 -> Average S2X SNR Calculator/3(scg_signal)
  Constant/1 -> Average S2X SNR Calculator/1(fs)
  " "/1 -> Switch/2
  Constant1/1 -> Switch/3
  r_pos/1 -> Switch/1

== system WorkingModel/SCG Analysis/Enabled SCG Analysis Subsystem/All Signals Signal Metric Characterization/SCG S2 3DMechAxis Signal Metric Characterization/Average Signal-to-Noise Ratio Calculator/Average S1 Signal-to-Noise Ratio ==
  r_pos : Inport
  scg_signal : Inport  Port=2
  " " : Constant  Value=s1snr_flag
  Average S1 SNR Calculator : MATLAB Function  TreatAsAtomicUnit=on
  Constant : Constant  Value=fs
  Constant1 : Constant  Value=0
  Switch : Switch  Criteria=u2 > Threshold  AllowDiffInputSizes=on  SaturateOnIntegerOverflow=off  InputSameDT=off
  average_s1snr : Outport
  wires:
  Constant1/1 -> Switch/3
  r_pos/1 -> Switch/1
  Switch/1 -> Average S1 SNR Calculator/2(r_pos)
  " "/1 -> Switch/2
  Constant/1 -> Average S1 SNR Calculator/1(fs)
  Average S1 SNR Calculator/1(average_s1_snr) -> average_s1snr/1
  scg_signal/1 -> Average S1 SNR Calculator/3(scg_signal)

== system WorkingModel/SCG Analysis/Enabled SCG Analysis Subsystem/All Signals Signal Metric Characterization/SCG S2 3DMechAxis Signal Metric Characterization/Average Signal-to-Noise Ratio Calculator/Average S1X Signal-to-Noise Ratio ==
  r_pos : Inport
  scg_signal : Inport  Port=2
  " " : Constant  Value=s1xsnr_flag
  Average S1 SNR Amplitude Calculator : MATLAB Function  TreatAsAtomicUnit=on
  Constant : Constant  Value=fs
  Constant1 : Constant  Value=0
  Switch : Switch  Criteria=u2 > Threshold  AllowDiffInputSizes=on  SaturateOnIntegerOverflow=off  InputSameDT=off
  average_s1Xsnr : Outport
  wires:
  r_pos/1 -> Switch/1
  Constant1/1 -> Switch/3
  " "/1 -> Switch/2
  Constant/1 -> Average S1 SNR Amplitude Calculator/1(fs)
  scg_signal/1 -> Average S1 SNR Amplitude Calculator/3(scg_signal)
  Switch/1 -> Average S1 SNR Amplitude Calculator/2(r_pos)
  Average S1 SNR Amplitude Calculator/1(average_s1x_snr) -> average_s1Xsnr/1
